simulink model "A_EinfachesSubsys"  (R2018b)
settings: Solver=VariableStepAuto  StartTime=0.0  StopTime=5  MaxStep=0.1  RelTol=1e-3  EnableMultiTasking=on
model workspace (MAT data in the model file):
  AFS = 30
  AS = 0.5
  DT = 5
  cw = 1.3
  g = 9.81
  h0 = 500
  h1 = 150
  m = 85
  rho = 1.2
  v0 = 0
settings Model: Creator=Reichl  LastModifiedBy=Reichl
settings DataIOCC: SaveFormat=Array  OutputSaveName=h
settings OptimizationCC: LifeSpan=inf
settings DebuggingCC: SolverPrmCheckMsg=warning  SFUnexpectedBacktrackingDiag=warning  SFNoUnconditionalDefaultTransitionDiag=warning  SFExecutionAtInitializationDiag=none
settings HardwareCC: ProdBitPerPointer=32  ProdBitPerSizeT=32  ProdBitPerPtrDiffT=32  ProdLargestAtomicFloat=None  ProdIntDivRoundTo=Undefined  ProdEndianess=Unspecified  ProdWordSize=32  ProdHWDeviceType=32-bit Generic
settings ModelReferenceCC: PropagateSignalLabelsOutOfModel=off
settings SFSimCC: SimUseLocalCustomCode=off
settings RTWCC: RTWUseLocalCustomCode=off
settings CodeAppCC: StateflowObjectComments=on
settings GRTTargetCC: TargetLangStandard=C89/C90 (ANSI)  GeneratePreprocessorConditionals=Disable all
settings ConfigComp: CovMetricSettings=dw  CovHtmlReporting=on  CovSaveCumulativeToWorkspaceVar=on  CovSaveSingleToWorkspaceVar=on  CovExternalEMLEnable=off  CovSFcnEnable=off

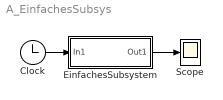
== system A_EinfachesSubsys ==
  Clock : Clock
  "EinfachesSubsystem " : Subsystem  TreatAsAtomicUnit=on
  Scope : Scope
  wires:
  Clock/1 -> "EinfachesSubsystem "/1(In1)
  "EinfachesSubsystem "/1(Out1) -> Scope/1

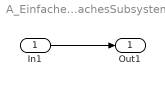
== system A_EinfachesSubsys/EinfachesSubsystem  ==
  In1 : Inport
  Out1 : Outport  InitialOutput=1.5
  wires:
  In1/1 -> Out1/1
